simulink model "Drehteller"  (R2022a)
settings: Solver=ode3  StartTime=0.0  StopTime=10.0  FixedStep=0.01  RelTol=1e-3  EnableMultiTasking=on
values from neighbouring files (symbols this model uses):
  A = 5    [Parametriesierung.m]
  I = 0.5    [Parametriesierung.m]
  igetr = 1080    [Parametriesierung.m]
  K = 8    [Parametriesierung.m]
  MRK = 1    [Parametriesierung.m]
  PHI = 0.001    [Parametriesierung.m]
  Ra = 40    [Parametriesierung.m]
  U = 24    [Parametriesierung.m]
settings Model: Creator=60251  LastModifiedBy=yufu
settings SolverCC: AlgebraicLoopSolver=TrustRegion
settings DebuggingCC: UnconnectedInputMsg=warning  UnconnectedOutputMsg=warning  UnconnectedLineMsg=warning  SFMachineParentedDataDiag=warning
settings RTWCC: DLArmComputeVersion=19.05

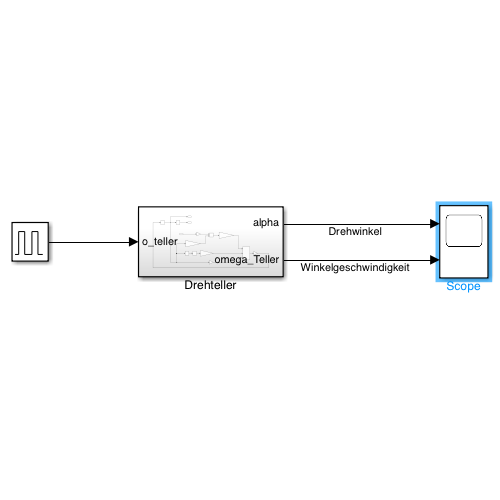
[thumbnail: Simulink's stored preview of the top-level diagram]
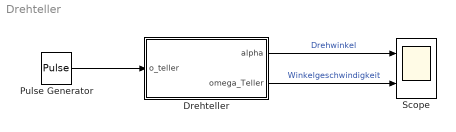
== system Drehteller ==
  Drehteller : Subsystem
  Pulse Generator : DiscretePulseGenerator  PulseType=Time based  PulseWidth=50
  Scope : Scope  NumInputPorts=2
  wires:
  Drehteller/1(alpha) -> Scope/1  "Drehwinkel"
  Drehteller/2(omega_Teller) -> Scope/2  "Winkelgeschwindigkeit"
  Pulse Generator/1 -> Drehteller/1(o_teller)

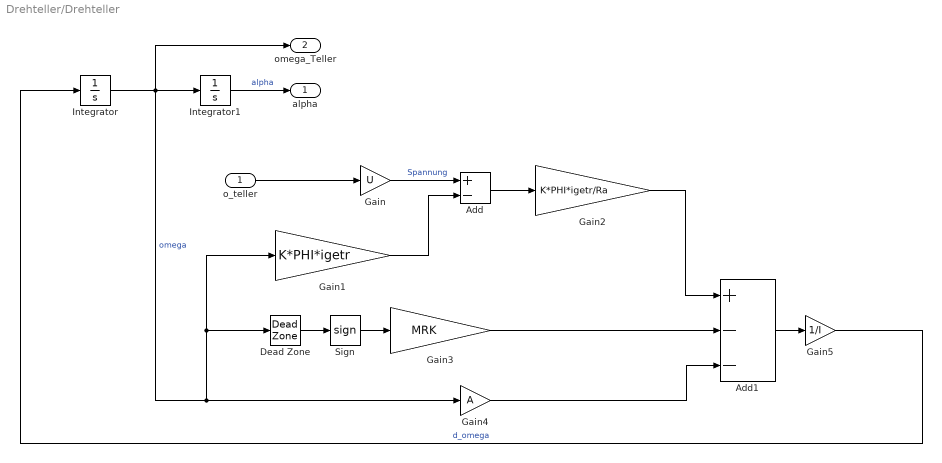
== system Drehteller/Drehteller ==
  o_teller : Inport
  Add : Sum  Inputs=+-
  Add1 : Sum  Inputs=+--
  Dead Zone : DeadZone
  Gain : Gain  Gain=U
  Gain1 : Gain  Gain=K*PHI*igetr
  Gain2 : Gain  Gain=K*PHI*igetr/Ra
  Gain3 : Gain  Gain=MRK
  Gain4 : Gain  Gain=A
  Gain5 : Gain  Gain=1/I
  Integrator : Integrator
  Integrator1 : Integrator
  Sign : Signum
  alpha : Outport
  omega_Teller : Outport  Port=2
  wires:
  o_teller/1 -> Gain/1
  Gain/1 -> Add/1  "Spannung"
  Integrator/1 -> omega_Teller/1, Integrator1/1, Gain4/1, Gain1/1, Dead Zone/1  "omega"
  Gain5/1 -> Integrator/1  "d_omega"
  Integrator1/1 -> alpha/1  "alpha"
  Gain1/1 -> Add/2
  Add/1 -> Gain2/1
  Sign/1 -> Gain3/1
  Dead Zone/1 -> Sign/1
  Gain2/1 -> Add1/1
  Gain3/1 -> Add1/2
  Gain4/1 -> Add1/3
  Add1/1 -> Gain5/1
